simulink model "genericAW_atta"  (R2015a)
settings: Solver=ode5  SolverMode=SingleTasking  StartTime=0.0  StopTime=tstop  FixedStep=tstep  RelTol=1e-3  AbsTol=1e-6
values from neighbouring files (symbols this model uses):
  Ac = rlqg.A    [atta_sim.m]
  Ap = A    [atta_sim.m]
  AW = AWfull    [atta_sim.m]    (also in fullorder_ctf.m = ss(Ap+Bp*F,Bp,[F; Cp+Dp*F],[zeros(m,m); Dp]))
  baru = ubar    (= 0.5)    [atta_sim.m]
  Bc = rlqg.B    [atta_sim.m]
  Bp = B    [atta_sim.m]
  Bpd = H    [atta_sim.m]
  Cc = rlqg.C    [atta_sim.m]
  Cp = C    [atta_sim.m]
  Dc = rlqg.D    [atta_sim.m]
  Dp = zeros(1,2)    [atta_sim.m]
  Dpd = zeros(1,1)    [atta_sim.m]
  p = size(Cp,1)    [fullorder_ctf.m]
undefined symbols (not defined in the file or in its folder): m, nd
libraries: simulink x1
settings Model: ExtModeTrigMode=oneshot  ExtModeArmWhenConnect=off  ExtModeAutoUpdateStatusClock=off  Creator=mct6  LastModifiedBy=mct6
settings DataIOCC: LimitDataPoints=off  SignalLoggingSaveFormat=ModelDataLogs  SaveOutput=off  SignalLoggingName=sigsOut
settings OptimizationCC: BooleanDataType=off  InitFltsAndDblsToZero=on
settings DebuggingCC: AlgebraicLoopMsg=none  SaveWithParameterizedLinksMsg=none  UnderspecifiedInitializationDetection=Classic  MergeDetectMultiDrivingBlocksExec=none  SignalResolutionControl=TryResolveAllWithWarning  MultiTaskDSMMsg=warning  MultiTaskCondExecSysMsg=none  FcnCallInpInsideContextMsg=UseLocalSettings
settings HardwareCC: TargetUnknown=on
settings GRTTargetCC: TargetFcnLib=ansi_tfl_tmw.mat  ModelReferenceCompliant=off  CombineOutputUpdateFcns=off  MatFileLogging=off  GRTInterface=on

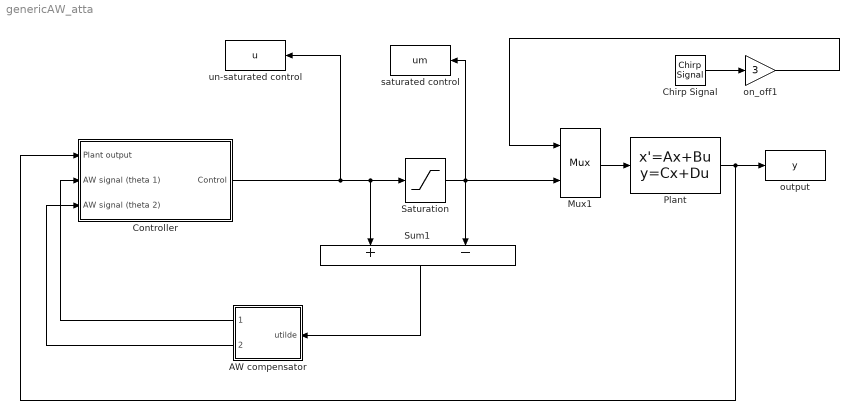
== system genericAW_atta ==
  AW compensator : Subsystem
  Chirp Signal : simulink/Sources/Chirp Signal  f1=0.1  T=14  f2=140
  Controller : Subsystem
  Mux1 : Mux  Inputs=[nd m]
  Plant : StateSpace  A=Ap  B=[Bpd Bp]  C=Cp  D=[Dpd Dp]  X0=0
  Saturation : Saturate  UpperLimit=baru  LowerLimit=-baru
  Sum1 : Sum  Inputs=+-  SaturateOnIntegerOverflow=on  InputSameDT=on  OutDataTypeStr=Inherit: Same as first input
  on_off1 : Gain  Gain=3
  output : ToWorkspace  VariableName=y  SaveFormat=Structure With Time  SampleTime=-1
  saturated control : ToWorkspace  VariableName=um  SaveFormat=Structure With Time  SampleTime=-1
  un-saturated control : ToWorkspace  VariableName=u  SaveFormat=Structure With Time  SampleTime=-1
  wires:
  Controller/1(Control) -> Saturation/1, Sum1/1, un-saturated control/1
  Plant/1 -> output/1, Controller/1(Plant output)
  Saturation/1 -> Sum1/2, Mux1/2, saturated control/1
  Sum1/1 -> AW compensator/1(utilde)
  AW compensator/2(theta 2) -> Controller/3(AW signal (theta 2))
  AW compensator/1(theta 1) -> Controller/2(AW signal (theta 1))
  Mux1/1 -> Plant/1
  on_off1/1 -> Mux1/1
  Chirp Signal/1 -> on_off1/1

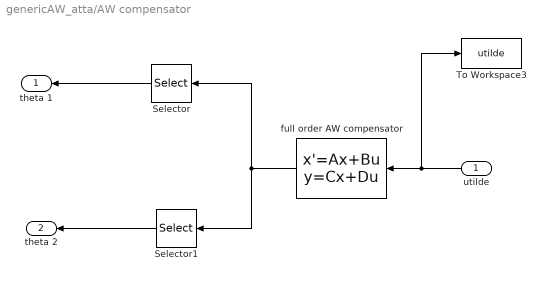
== system genericAW_atta/AW compensator ==
  utilde : Inport
  Selector : Selector  InputPortWidth=m+p  Indices=[1:m]
  Selector1 : Selector  InputPortWidth=m+p  Indices=[m+1:m+p]
  To Workspace3 : ToWorkspace  VariableName=utilde  SaveFormat=Structure With Time  SampleTime=-1
  full order AW compensator : StateSpace  A=AW.a  B=AW.b  C=AW.c  D=AW.d  X0=0
  theta 1 : Outport  InitialOutput=0
  theta 2 : Outport  Port=2  InitialOutput=0
  wires:
  utilde/1 -> full order AW compensator/1, To Workspace3/1
  full order AW compensator/1 -> Selector/1, Selector1/1
  Selector/1 -> theta 1/1
  Selector1/1 -> theta 2/1

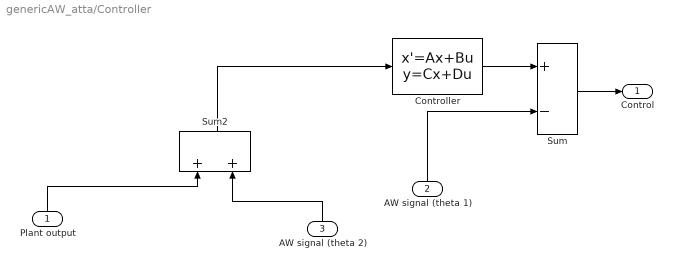
== system genericAW_atta/Controller ==
  Plant output : Inport
  AW signal (theta 1) : Inport  Port=2
  AW signal (theta 2) : Inport  Port=3
  Controller : StateSpace  A=Ac  B=Bc  C=Cc  D=Dc  X0=0
  Sum : Sum  Inputs=+-  SaturateOnIntegerOverflow=on  InputSameDT=on  OutDataTypeStr=Inherit: Same as first input
  Sum2 : Sum  SaturateOnIntegerOverflow=on  InputSameDT=on  OutDataTypeStr=Inherit: Same as first input
  Control : Outport
  wires:
  Sum2/1 -> Controller/1
  Plant output/1 -> Sum2/1
  Controller/1 -> Sum/1
  Sum/1 -> Control/1
  AW signal (theta 1)/1 -> Sum/2
  AW signal (theta 2)/1 -> Sum2/2
